simulink model "princessmodel2"  (R2013b)
settings: Solver=ode3  SolverMode=SingleTasking  StartTime=0.0  StopTime=inf  RelTol=1e-3
PreLoadFcn:
  | Ts = 0.1;
libraries: legonxtlib x5
settings Model: ExtModeTrigDuration=2  Creator=scastro  LastModifiedBy=grouleau
settings OptimizationCC: OptimizeModelRefInitCode=on  LifeSpan=1
settings DebuggingCC: SolverPrmCheckMsg=none  StateNameClashWarn=warning
settings HardwareCC: ProdLargestAtomicInteger=Long  ProdLargestAtomicFloat=Float  ProdEndianess=LittleEndian  ProdHWDeviceType=ARM Compatible->ARM 7
settings RTWCC: SystemTargetFile=realtime.tlc  GenerateMakefile=off  TemplateMakefile=realtime.tmf  Description=Run on Target Hardware  RTWVerbose=off  ProcessScript=realtime_make_rtw_hook
settings STFCustomTargetCC: TargetLibSuffix=.a  GenerateSampleERTMain=on  ERTCustomFileBanners=on  SupportNonInlinedSFcns=off  SupportVariableSizeSignals=on  MATLABClassNameForMDSCustomization=Simulink.SoftwareTarget.ERTCustomization  GRTInterface=off  SystemTargetFile=realtime.tlc
settings ERTTargetCC: CodeReplacementLibrary=ANSI_C  GenerateSampleERTMain=on  ParMdlRefBuildCompliant=off  CompOptLevelCompliant=off  ConcurrentExecutionCompliant=off  CombineOutputUpdateFcns=off  ERTFirstTimeCompliant=off  SupportContinuousTime=on  SupportVariableSizeSignals=on  ModelStepFunctionPrototypeControlCompliant=off  CPPClassGenCompliant=off  ExtModeTransport=1  ExtModeMexFile=ext_serial_win32_comm_no_acks_rtt_byteswap  ExtModeMexArgs=0 1 9600  InlinedParameterPlacement=NonHierarchical  ERTSrcFileBannerTemplate=realtime_code_template.cgt  ERTHdrFileBannerTemplate=realtime_code_template.cgt  ERTDataSrcFileTemplate=realtime_code_template.cgt  ERTDataHdrFileTemplate=realtime_code_template.cgt  ERTCustomFileTemplate=realtime_file_process.tlc

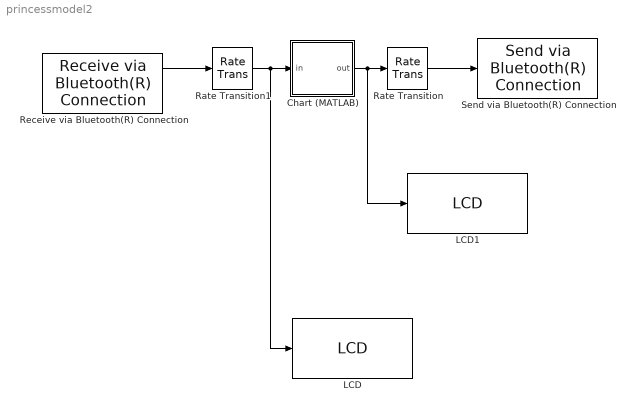
== system princessmodel2 ==
  Chart (MATLAB) : Stateflow chart  TreatAsAtomicUnit=on
  LCD : legonxtlib/LCD  slcdStr=In  slcdLine=1  slcdFormat=Decimal
  LCD1 : legonxtlib/LCD  slcdStr=Out  slcdLine=2  slcdFormat=Decimal
  Rate Transition : RateTransition  OutPortSampleTime=Ts
  Rate Transition1 : RateTransition  OutPortSampleTime=0.004
  Receive via Bluetooth(R) Connection : legonxtlib/Receive via Bluetooth(R) Connection  mailbox=3  dataType=uint8  dataSize=1  sampleTime=Ts
  Send via Bluetooth(R) Connection : legonxtlib/Send via Bluetooth(R) Connection  mailbox=4
  wires:
  Receive via Bluetooth(R) Connection/1 -> Rate Transition1/1
  Chart (MATLAB)/1(out) -> LCD1/1, Rate Transition/1
  Rate Transition/1 -> Send via Bluetooth(R) Connection/1
  Rate Transition1/1 -> LCD/1, Chart (MATLAB)/1(in)

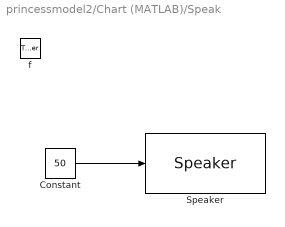
== system princessmodel2/Chart (MATLAB)/Speak ==
  f : TriggerPort  TriggerType=function-call
      settings: CopyFcn=Stateflow.SLINSF.SimulinkMan.removeBlockPreDeleteFcn  PreDeleteFcn=Stateflow.SLINSF.SimulinkMan.unsafePredeleteFcn
  Constant : Constant  Value=50
  Speaker : legonxtlib/Speaker  sinputMode=Volume only  sspeakerFreq=800  sspeakerVolume=50  sspeakerDuration=100
  wires:
  Constant/1 -> Speaker/1

== stateflow chart princessmodel2/Chart (MATLAB) ==
  state Wait
  state s1
    entry: Speak;
  state Speak [function]
  state s2
    en:out=uint8(22);
    Speak
  state s3
    en:Speak
  state s9
    en:out=uint8(23);
    Speak
  (default) -> Wait
  s9 -> Wait
  Wait -> s1 : [isequal(in,uint8(11))]
  s1 -> s2 : after(5, sec)
  s2 -> s3 : [isequal(in,uint8(12))]
  s3 -> s9 : after(5, sec)
  data: in input; out output
